simulink model "USRP_Rx"  (R2020a)
settings: Solver=FixedStepAuto  StartTime=0.0  StopTime=3  RelTol=1e-3
StopFcn:
  | I = real(data);
  | Q = imag(data);
values from neighbouring files (symbols this model uses):
  data = zeros(ceil(n/27),16)    [IMU_ADI_read.m]    (also in IMU_SBG_read.m = zeros(n,12); IMU_read.m; MTi_parse.m = fread(fileID, Inf, 'uint8=>uint8'); SBG_imu_read.m = zeros(n,12))
libraries: commsdrhw_v2 x1
settings Model: SimulationMode=rapid-accelerator  Creator=longt  LastModifiedBy=longt
settings DataIOCC: SaveOutput=off  SignalLogging=off  DSMLogging=off  SaveTime=off  ReturnWorkspaceOutputs=off

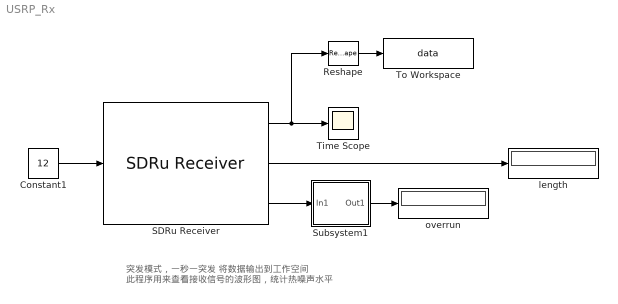
== system USRP_Rx ==
  note: 突发模式，一秒一突发
      | 将数据输出到工作空间
      | 此程序用来查看接收信号的波形图，统计热噪声水平
  Constant1 : Constant  Value=12
  Reshape : Reshape  OutputDimensionality=Column vector (2-D)
  SDRu Receiver : commsdrhw_v2/SDRu Receiver  rxtx=rx  initializeIPAddress=0  devMap=10  USRP2_IP=192.168.10.2  USRP_IP_X300=192.168.10.2  USRP_IP_X310=No devices found  USRP_IP_N300=192.168.10.2  USRP_IP_N310=192.168.10.2  USRP_IP_N320=192.168.10.2  USRP_serialNumB200=No devices found  USRP_serialNumB210=315F337  platform=B210  prevPlatform=B210  lastIPAddressPopup=192.168.10.2  USRP_ID=315F337  LastIPAddress=192.168.10.2  IsTwinRXDaughterboard=off  EnableTwinRXPhaseSync=off  losrc=0  ChannelMapping=1  centerFrequencySrc=Dialog  centerFrequency=1575.42e6  loOffsetSrc=Dialog  loOffset=0  gainSrc=Input port  gain=32  PPSSource=Internal  clockSource=Internal  masterClkRateParam=16000000  masterClkRateB200=32e6  masterClkRateB210=16e6  masterClkRateX300=200e6  masterClkRateX310=200e6  masterClkRateN300=125e6  masterClkRateN310=125e6  masterClkRateN320=200e6  masterClkRate=100e6  masterClkRateTwinRX=200e6  decimInterpSrc=Dialog  decimInterpPort=512  lastDecimSource=Dialog  decimInterp=4  USRP2_IP_NUM=[51 49 53 70 51 51 55]  sampleRate=4000000  sampleTime=2.5e-07  TransportDataType=int16  overrunUnderrunPort=on  outputDatatype=Same as transport data type  frameLength=4000  HOST_DATA_PORT=0  HOST_CONTROL_PORT=0  USRP2_DATA_PORT=0  USRP2_CONTROL_PORT=0  bufferMode=Continuous streaming  EnableBurstMode=on  NumFramesInBurst=1000
      settings: SourceProductBaseCode=USRP
  Subsystem1 : Subsystem
  Time Scope : Scope
  To Workspace : ToWorkspace  VariableName=data  SampleTime=-1
      settings: Save2DSignal=2-D array (concatenate along first dimension)
  length : Display
  overrun : Display
  wires:
  SDRu Receiver/3 -> Subsystem1/1(In1)
  Subsystem1/1(Out1) -> overrun/1
  Constant1/1 -> SDRu Receiver/1
  SDRu Receiver/1 -> Reshape/1, Time Scope/1
  SDRu Receiver/2 -> length/1
  Reshape/1 -> To Workspace/1

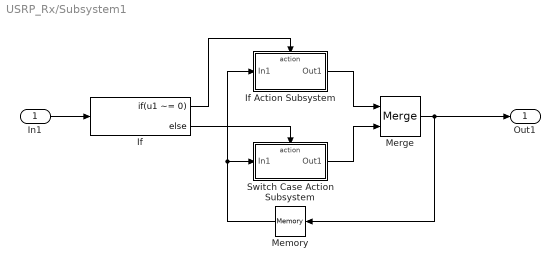
== system USRP_Rx/Subsystem1 ==
  In1 : Inport
  If : If  IfExpression=u1 ~= 0
  If Action Subsystem : Subsystem  TreatAsAtomicUnit=on
  Memory : Memory
  Merge : Merge
  Switch Case Action Subsystem : Subsystem  TreatAsAtomicUnit=on
  Out1 : Outport  VectorParamsAs1DForOutWhenUnconnected=off
  wires:
  If/2 -> Switch Case Action Subsystem/Action
  If/1 -> If Action Subsystem/Action
  In1/1 -> If/1
  Memory/1 -> If Action Subsystem/1(In1), Switch Case Action Subsystem/1(In1)
  Merge/1 -> Memory/1, Out1/1
  If Action Subsystem/1(Out1) -> Merge/1
  Switch Case Action Subsystem/1(Out1) -> Merge/2

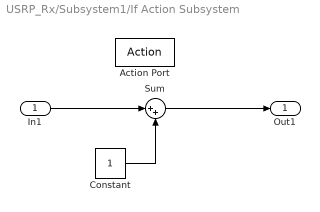
== system USRP_Rx/Subsystem1/If Action Subsystem ==
  In1 : Inport
  Action Port : ActionPort  ActionPortLabel=if(u1 ~= 0)
  Constant : Constant
  Sum : Sum  Inputs=|++
  Out1 : Outport  VectorParamsAs1DForOutWhenUnconnected=off
  wires:
  Constant/1 -> Sum/2
  In1/1 -> Sum/1
  Sum/1 -> Out1/1

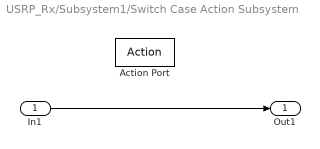
== system USRP_Rx/Subsystem1/Switch Case Action Subsystem ==
  In1 : Inport
  Action Port : ActionPort  ActionPortLabel=else
  Out1 : Outport  VectorParamsAs1DForOutWhenUnconnected=off
  wires:
  In1/1 -> Out1/1
